simulink model "sst_llc_npc_inv"  (R2025b)
settings: Solver=ode23tb  StartTime=0.0  StopTime=simlength  FixedStep=tc  MaxStep=tc
values from neighbouring files (symbols this model uses):
  Adrso = eye(2) + Arso*ts_inv    [init_model.m]
  Aresd_max = eye(2) + Ares_max*ts_afe    [init_model.m]
  Aresd_min = eye(2) + Ares_min*ts_afe    [init_model.m]
  Aresd_nom = eye(2) + Ares_nom*ts_afe    [init_model.m]
  Bresd = Bres*ts_afe    [init_model.m]
  CFi_dc2 = 900e-6*4    (= 0.0036)    [init_model.m]
  Cresd = Cres    [init_model.m]
  Crso = [1 0]    [init_model.m]
  delta = 0.025    [init_model.m]
  fPWM_DAB = fPWM*4    (= 20000)    [init_model.m]
  fPWM_LLC_pu = 0.54    [init_model.m]
  freq = f_grid    [init_model.m]
  Iac_FS = I_phase_normalization_factor    [init_model.m]
  Idc_FS = max(Idab1_dc_nom,Idab2_dc_nom) * margin_factor    [init_model.m]
  iph_grid_pu_ref = 2.75    [init_model.m]
  ki_afe = 18    [init_model.m]
  ki_pll = 3140    [init_model.m]
  ki_rpi = 18    [init_model.m]
  kp_afe = 0.25    [init_model.m]
  kp_pll = 314    [init_model.m]
  kp_rpi = 0.25    [init_model.m]
  Ldrso = acker(Adrso',Crso',polesdrso)'    [init_model.m]
  LFu1_AFE = 0.33e-3    (= 0.00033)    [init_model.m]
  n_modules = 2    [init_model.m]
  RLFu1_AFE = 157*0.05*LFu1_AFE    (= 0.0025905)    [init_model.m]
  tc = ts_dab/100    (= 5e-07)    [init_model.m]
  ts_afe = 1/fPWM_AFE    (= 0.0002)    [init_model.m]
  ts_dab = 1/fPWM_DAB    (= 5e-05)    [init_model.m]
  ts_inv = 1/fPWM_INV    (= 0.0002)    [init_model.m]
  Vac_FS = V_phase_normalization_factor    [init_model.m]
  Vdab2_dc_nom = 750    [init_model.m]
  Vdc_FS = max(Vdab1_dc_nom,Vdab2_dc_nom) * margin_factor    [init_model.m]
undefined symbols (not defined in the file or in its folder): f_grid, Ld2_trafo, omega_grid_nom, Rd2_trafo, V_phase_normalization_factor
libraries: fl_lib x67, nesl_utility x39, full_bridge_mosfet_based_with_thermal_model x4, full_bridge_mosfet_based_with_thermal_model_zvs x4, pi_ctrl x4, discrete_time_low_pass_filter x4, full_bridge_three_level_npc_ideal_switch_based_model x3, single_phase_transformer x2, moving_average_filter x2, resonant_llc_modulator x2, full_bridge_ideal_switch x2, dclink_for_three_levels x2
(part 1 of 4)
settings Model: SimulationMode=accelerator  Creator=LTNBDA  LastModifiedBy=dbagn
settings SolverCC: ZeroCrossControl=EnableAll  ZeroCrossAlgorithm=Adaptive  AlgebraicLoopSolver=TrustRegion  SolverResetMethod=Robust  AutoInsertRateTranBlk=on
settings DataIOCC: LimitDataPoints=on  MaxDataPoints=1  SaveFormat=Array  SignalLoggingSaveFormat=ModelDataLogs  SaveOutput=off  SignalLogging=off  DSMLogging=off  SaveTime=off  ReturnWorkspaceOutputs=off
settings OptimizationCC: ExpressionDepthLimit=2147483647.0  InitFltsAndDblsToZero=on  EfficientMapNaN2IntZero=off  LifeSpan=inf
settings DebuggingCC: SaveWithParameterizedLinksMsg=none  UnderspecifiedInitializationDetection=Classic  MergeDetectMultiDrivingBlocksExec=none  SignalResolutionControl=TryResolveAllWithWarning  SolverPrmCheckMsg=warning  MultiTaskDSMMsg=warning  MultiTaskCondExecSysMsg=none  MultiTaskRateTransMsg=warning  FcnCallInpInsideContextMsg=warning  StateNameClashWarn=warning  SFUnexpectedBacktrackingDiag=warning  SFNoUnconditionalDefaultTransitionDiag=warning  ArithmeticOperatorsInVariantConditions=warning
settings HardwareCC: ProdBitPerLong=64.0  ProdLargestAtomicFloat=None  ProdIntDivRoundTo=Undefined  ProdEndianess=Unspecified  ProdHWDeviceType=Generic->64-bit Embedded Processor (LP64)  TargetBitPerPointer=64.0  TargetBitPerSizeT=64.0  TargetBitPerPtrDiffT=64.0  TargetLongLongMode=on  TargetIntDivRoundTo=Zero  TargetEndianess=LittleEndian  TargetWordSize=64.0  TargetHWDeviceType=MATLAB Host  ProdEqTarget=off
settings ModelReferenceCC: EnableRefExpFcnMdlSchedulingChecks=on  PropagateSignalLabelsOutOfModel=off
settings SFSimCC: SimUseLocalCustomCode=off  CustomCodeUndefinedFunction=UseInterfaceOnly
settings SFSimCC: SimCustomHeaderCode=|
  | #include "rpi.h"
  | #include "rpi_simulink.h"
  | #include "mavgflt.h"
  | #include "mavgflt_simulink.h"
  | #include "bemf_obsv.h"
  | #include "bemf_obsv_simulink.h"
  | #include "bemf_obsv_load_est.h"
  | #include "bemf_obsv_load_est_simulink.h"
  | #include "dqvector_pi.h"
  | #include "dqvector_pi_simulink.h"
  | #include "sv_pwm_simulink.h"
  | #include "sv_pwm.h"
  | #include "first_harmonic_tracker.h"
  | #include "first_harmonic_tracker_simulink.h"
  | #include "dqpll_thyr.h"
  | #include "dqpll_thyr_simulink.h"
  | #include "dqpll_grid.h"
  | #include "dqpll_grid_simulink.h"
settings SFSimCC: SimUserSources=|
  | "mavgflt_simulink.c"
  | "mavgflt.c"
  | "bemf_obsv_simulink.c"
  | "bemf_obsv.c"
  | "bemf_obsv_load_est_simulink.c"
  | "bemf_obsv_load_est.c"
  | "dqvector_pi.c"
  | "dqvector_pi_simulink.c"
  | "sv_pwm_simulink.c"
  | "sv_pwm.c"
  | "first_harmonic_tracker_simulink.c"
  | "first_harmonic_tracker.c"
  | "dqpll_thyr_simulink.c"
  | "dqpll_thyr.c"
  | "dqpll_grid_simulink.c"
  | "dqpll_grid.c"
  | "rpi_simulink.c"
  | "rpi.c"
settings SFSimCC: SimUserIncludeDirs=|
  | include
  | src
settings RTWCC: RTWUseLocalCustomCode=off  GPUComputeCapability=3.5
settings CodeAppCC: MaxIdLength=128.0  StateflowObjectComments=on
settings GRTTargetCC: TargetLangStandard=C89/C90 (ANSI)  CombineOutputUpdateFcns=off  GRTInterface=on
settings ConfigComp: CovMetricSettings=dw  CovSaveCumulativeToWorkspaceVar=on  CovSaveSingleToWorkspaceVar=on  CovExternalEMLEnable=off
settings SimscapeCC: SimscapeNormalizeSystem=off

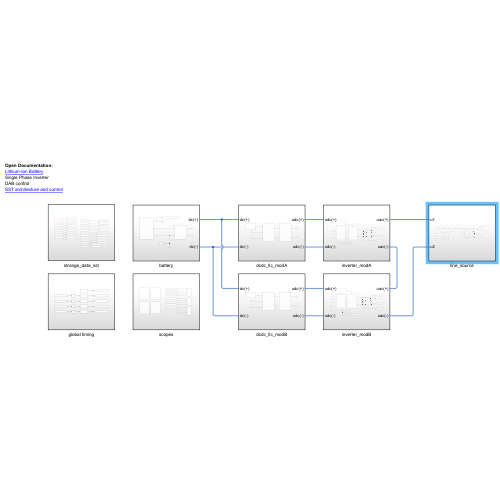
[thumbnail: Simulink's stored preview of the top-level diagram]
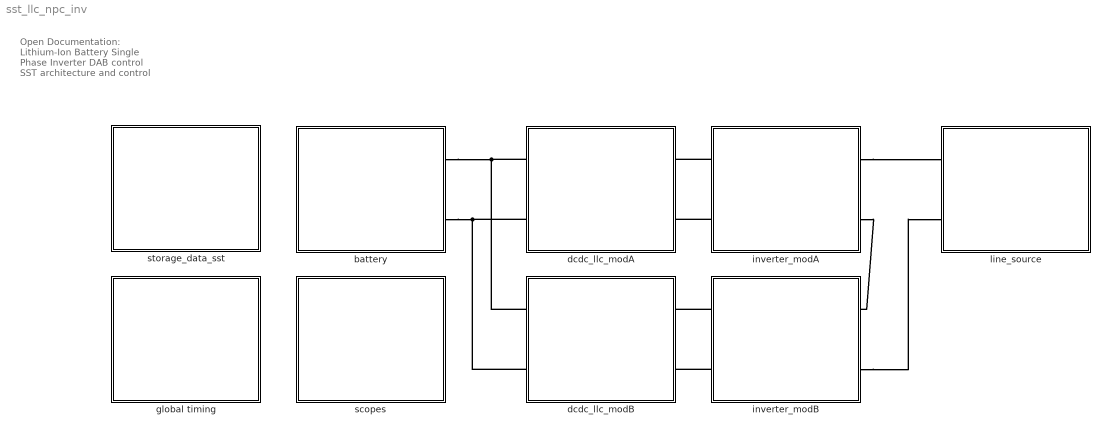
== system sst_llc_npc_inv ==
  note: Open Documentation:
      | Lithium-Ion Battery
      | Single Phase Inverter
      | DAB control
      | SST architecture and control
  battery : Subsystem
  dcdc_llc_modA : Subsystem
  dcdc_llc_modB : Subsystem
  global timing : Subsystem
  inverter_modA : Subsystem
  inverter_modB : Subsystem
  line_source : Subsystem
  scopes : Subsystem
  storage_data_sst : Subsystem
  connections:
  inverter_modA/LConn2 -- dcdc_llc_modA/RConn2
  inverter_modA/LConn1 -- dcdc_llc_modA/RConn1
  battery/RConn1 -- dcdc_llc_modB/LConn1 -- dcdc_llc_modA/LConn1
  battery/RConn2 -- dcdc_llc_modB/LConn2 -- dcdc_llc_modA/LConn2
  inverter_modB/LConn1 -- dcdc_llc_modB/RConn1
  inverter_modB/LConn2 -- dcdc_llc_modB/RConn2
  inverter_modA/RConn1 -- line_source/LConn1
  inverter_modA/RConn2 -- inverter_modB/RConn1
  inverter_modB/RConn2 -- line_source/LConn2

== system sst_llc_npc_inv/battery ==
  Electrical Reference1 : fl_lib/Electrical/Electrical Elements/Electrical Reference
  Solver Configuration : nesl_utility/Solver Configuration  PhysicalDomain=network_engine_domain  SubClassName=solver  LeftPortType=input  RightPortType=generic  Tones=[]  Harmonics=[]  SimulateNoise=off  Profile=off  UseLocalSampling=off  EnableSwitchedLinearOptims=on  FrequencyDomain=off  UseCCode=off  RelTol=0.001  AbsTol=0.001  MinStep=1e-09  ToWorkspace=off  RevertToSquareIcSolve=off  NumHomotopyIterations=100  PhasorMode=off  PhasorModeNumHarmonics=1  ConsistencySolver=NEWTON_FTOL  IndexReductionMethod=DerivativeReplacement  DoDC=on  ResidualTolerance=1e-09  ConsistencyTolSource=GLOBAL  ConsistencyAbsTol=0.001  ConsistencyRelTol=0.001  ConsistencyTolFactor=0.001  UseLocalSolver=on  LocalSolverChoice=NE_BACKWARD_EULER_ADVANCER  ResolveIndetEquations=on  FunctionEvalNumThread=1  LocalSolverSampleTime=tc  DoFixedCost=on  MaxNonlinIter=5  MaxModeIter=2  ComputeImpulses=off  ImpulseIterations=2  LinearAlgebra=auto  LinearAlgebraNumThread=0  EquationFormulation=NE_TIME_EF  DelaysMemoryBudget=1024  AutomaticFiltering=on  FilteringTimeConstant=0.001  PartitionStorageMethod=AS_NEEDED  PartitionMemoryBudget=1024  PartitionMethod=ROBUST  MultibodyUseLocalSolver=off  MultibodyLocalSolverChoice=ODE1  MultibodyLocalSolverSampleTime=0.001
  To Workspace14 : ToWorkspace  VariableName=battery_data  SampleTime=tc
      settings: MaxDataPoints=Nc
  litium ion battery : Scope
      settings: ActiveDisplayYMinimum=-797.80832786516225  ActiveDisplayYMaximum=1570.6184440426914  DataLoggingVariableName=ScopeData3
  litium_ion_battery : litium_ion_battery/litium_ion_battery  Q=Q  number_of_cells=number_of_cells  E_1=E_1  E0=E0  E1=E1  E2=E2  E3=E3  Elog=Elog  R0=R0  R1=R1  C1=C1  M=M  alpha=alpha  soc_init=0.85  ts_battery=ts_battery  q1Kalman=q1Kalman  q2Kalman=q2Kalman  q3Kalman=q3Kalman  rKalman=rKalman  tc=tc
  single_phase_ui_measure : Subsystem
  dc(+) : PMIOPort  Side=Right
  dc(-) : PMIOPort  Port=2  Side=Right
  wires:
  litium_ion_battery/1 -> To Workspace14/1, litium ion battery/1
  connections:
  litium_ion_battery/RConn2 -- single_phase_ui_measure/LConn2 -- Electrical Reference1/LConn1 -- Solver Configuration/RConn1
  single_phase_ui_measure/RConn1 -- dc(+)/RConn1
  single_phase_ui_measure/LConn1 -- litium_ion_battery/RConn1
  dc(-)/RConn1 -- single_phase_ui_measure/RConn2

== system sst_llc_npc_inv/dcdc_llc_modA ==
  dc/dc with galvanic isolation : Subsystem
  llc_ctrl : Subsystem
  ui_measure : Subsystem
  udc(+) : PMIOPort  Side=Right
  udc(-) : PMIOPort  Port=2  Side=Right
  dc(+) : PMIOPort  Port=3  Side=Left
  dc(-) : PMIOPort  Port=4  Side=Left
  wires:
  llc_ctrl/1(dab_gate_cmds) -> dc/dc with galvanic isolation/1(dab_gate_cmds)
  connections:
  dc/dc with galvanic isolation/RConn1 -- ui_measure/LConn1
  dc/dc with galvanic isolation/RConn2 -- ui_measure/LConn2
  udc(+)/RConn1 -- ui_measure/RConn1
  udc(-)/RConn1 -- ui_measure/RConn2
  dc(-)/RConn1 -- dc/dc with galvanic isolation/LConn2
  dc(+)/RConn1 -- dc/dc with galvanic isolation/LConn1

== system sst_llc_npc_inv/dcdc_llc_modB ==
  dc/dc with galvanic isolation : Subsystem
  llc_ctrl : Subsystem
  ui_measure : Subsystem
  udc(+) : PMIOPort  Side=Right
  udc(-) : PMIOPort  Port=2  Side=Right
  dc(+) : PMIOPort  Port=3  Side=Left
  dc(-) : PMIOPort  Port=4  Side=Left
  wires:
  llc_ctrl/1(dab_gate_cmds) -> dc/dc with galvanic isolation/1(dab_gate_cmds)
  connections:
  dc(+)/RConn1 -- dc/dc with galvanic isolation/LConn1
  dc(-)/RConn1 -- dc/dc with galvanic isolation/LConn2
  udc(-)/RConn1 -- ui_measure/RConn2
  udc(+)/RConn1 -- ui_measure/RConn1
  dc/dc with galvanic isolation/RConn2 -- ui_measure/LConn2
  dc/dc with galvanic isolation/RConn1 -- ui_measure/LConn1

== system sst_llc_npc_inv/global timing ==
  Unit Delay{,1..3} (4 alike) : UnitDelay  SampleTime=tc  HasFrameUpgradeWarning=on
  time_afe1 : Subsystem  mask{k=1}
      mask prompts: k "Time Gain"
      mask Display:
      | disp('time-gen');
      | port_label('input', 1, 'crt');
      | port_label('output', 1, 'tout');
  time_afe2 : Subsystem  mask{k=1}
      mask prompts: k "Time Gain"
      mask Display:
      | disp('time-gen');
      | port_label('input', 1, 'crt');
      | port_label('output', 1, 'tout');
  time_afe3 : Subsystem  mask{k=1}
      mask prompts: k "Time Gain"
      mask Display:
      | disp('time-gen');
      | port_label('output', 1, 'tout');
  time_inv1 : Subsystem  mask{k=1}
      mask prompts: k "Time Gain"
      mask Display:
      | disp('time-gen');
      | port_label('input', 1, 'crt');
      | port_label('output', 1, 'tout');
  time_inv2 : Subsystem  mask{k=1}
      mask prompts: k "Time Gain"
      mask Display:
      | disp('time-gen');
      | port_label('input', 1, 'crt');
      | port_label('output', 1, 'tout');
  tag scope: time_afe_module_1=global, time_afe_module_2=global, time_dab_module_1=global, time_dab_module_2=global, time_master=global
  wires:
  time_afe1/1(Out1) -> [time_afe_module_1]
  time_afe2/1(Out1) -> [time_dab_module_1]
  time_inv2/1(Out1) -> [time_dab_module_2]
  time_inv1/1(Out1) -> [time_afe_module_2]
  time_afe3/1(Out1) -> [time_master]
  [local_time_corr_afe1] -> Unit Delay/1
  Unit Delay/1 -> time_afe1/1(correction_time)
  [local_time_corr_dab1] -> Unit Delay1/1
  Unit Delay1/1 -> time_afe2/1(correction_time)
  [local_time_corr_afe2] -> Unit Delay2/1
  Unit Delay2/1 -> time_inv1/1(correction_time)
  Unit Delay3/1 -> time_inv2/1(correction_time)
  [local_time_corr_dab2] -> Unit Delay3/1

== system sst_llc_npc_inv/inverter_modA ==
  Bus Selector : BusSelector  OutputSignals=udc
  CFu_ac : fl_lib/Electrical/Electrical Elements/Capacitor  c=CFu_AFE F  r=RCFu_AFE Ohm  g=0 1/Ohm  i_specify=off  i_priority=None  i=0 A  i_nominal_specify=off  i_nominal_value=1  i_nominal_unit=A  v_specify=off  v_priority=None  v=0 V  v_nominal_specify=off  v_nominal_value=1  v_nominal_unit=V  vc_specify=off  vc_priority=High  vc=0 V  vc_nominal_specify=off  vc_nominal_value=1  vc_nominal_unit=V
  Current Sensor : fl_lib/Electrical/Electrical Sensors/Current Sensor
  Current Sensor1 : fl_lib/Electrical/Electrical Sensors/Current Sensor
  LFu_ac_1 : fl_lib/Electrical/Electrical Elements/Inductor  l=LFu1_AFE/2 H  r=RLFu1_AFE/2 Ohm  g=0 1/Ohm  i_specify=off  i_priority=None  i=0 A  i_nominal_specify=off  i_nominal_value=1  i_nominal_unit=A  v_specify=off  v_priority=None  v=0 V  v_nominal_specify=off  v_nominal_value=1  v_nominal_unit=V  i_L_specify=off  i_L_priority=High  i_L=0 A  i_L_nominal_specify=off  i_L_nominal_value=1  i_L_nominal_unit=A
  LFu_ac_2 : fl_lib/Electrical/Electrical Elements/Inductor  l=LFu1_AFE/2 H  r=RLFu1_AFE/2 Ohm  g=0 1/Ohm  i_specify=off  i_priority=None  i=0 A  i_nominal_specify=off  i_nominal_value=1  i_nominal_unit=A  v_specify=off  v_priority=None  v=0 V  v_nominal_specify=off  v_nominal_value=1  v_nominal_unit=V  i_L_specify=off  i_L_priority=High  i_L=0 A  i_L_nominal_specify=off  i_L_nominal_value=1  i_L_nominal_unit=A
  Open Circuit : fl_lib/Electrical/Electrical Elements/Open Circuit  v_specify=off  v_priority=None  v=0 V  v_nominal_specify=off  v_nominal_value=1  v_nominal_unit=V
  Resistor : fl_lib/Electrical/Electrical Elements/Resistor  R=10e3 Ohm  i_specify=off  i_priority=None  i=0 A  i_nominal_specify=off  i_nominal_value=1  i_nominal_unit=A  v_specify=off  v_priority=None  v=0 V  v_nominal_specify=off  v_nominal_value=1  v_nominal_unit=V
  Voltage Sensor1 : fl_lib/Electrical/Electrical Sensors/Voltage Sensor
  dclink : dclink_for_three_levels/dclink  Cdc1=CFi_dc2*2  Cdc2=CFi_dc2*2  Rudc_measure=107e3  Vdc_scale=Vdc_FS
  iph : nesl_utility/PS-Simulink Converter  PhysicalDomain=network_engine_domain  SubClassName=ps_output  LeftPortType=input  RightPortType=output  PseudoPeriodic=off  Frequencies=[]  VectorFormat=1-D array  Unit=A  AffineConversion=off
  single phase inverter : Subsystem
      settings: PortSchema="{\"entries\":[{\"content\":{\"sides\":[{\"content\":{\"connectorIds\":[\"LConn1\",\"LConn2\"]},\"type\":\"ConnectorPlacement.EquallySpacedRectSide\",\"uuid\":\"4fcf4fea-d38f-431b-8a91-be3ce9782faf\"},{\"content\":{\"connectorIds\":[\"RConn1\",\"RConn2\",\"RConn3\"],\"side\":\"RIGHT\"},\"type\":\"ConnectorPlacement.EquallySpacedRectSide\",\"uuid\":\"0aa56277-92e9-4e3b-84c7-43398254a4d8\"},{\"content\":{\"connectorIds\":[\"In1\"],\"side\":\"TOP\"},\"type\":\"ConnectorPlacement.EquallySpacedRectSide\",\"uuid\":\"5cd150dc-bcaf-4cd7-b2a8-3db203726730\"}]},\"type\":\"ConnectorPlacement.EquallySpacedConnector\",\"uuid\":\"bf8194c4-c327-4d40-bea4-f1e7617f80b4\"}],\"packageUris\":[\"http://schema.mathworks.com/mf0/Connector/R2020b\"],\"version\":\"1.0\"}"
  single phase inverter control1 : Subsystem
  uph1 : nesl_utility/PS-Simulink Converter  PhysicalDomain=network_engine_domain  SubClassName=ps_output  LeftPortType=input  RightPortType=output  PseudoPeriodic=off  Frequencies=[]  VectorFormat=1-D array  Unit=V  AffineConversion=off
  uph2 : nesl_utility/PS-Simulink Converter  PhysicalDomain=network_engine_domain  SubClassName=ps_output  LeftPortType=input  RightPortType=output  PseudoPeriodic=off  Frequencies=[]  VectorFormat=1-D array  Unit=A  AffineConversion=off
  uac(+) : PMIOPort  Side=Right
  uac(-) : PMIOPort  Port=2  Side=Right
  udc(+) : PMIOPort  Port=3  Side=Left
  udc(-) : PMIOPort  Port=4  Side=Left
  tag scope: CFu_ac_current_modA=global, dclink_inverter_modA=global, dclink_voltage_inverter_modA=global, inverter_current_output_modA=global, inverter_voltage_output_modA=global, u_ctrl_out_master=global
  wires:
  Bus Selector/1 -> [dclink_voltage_inverter_modA]  "<udc>"
  single phase inverter control1/1(gate_cmds) -> single phase inverter/1(gate_commands)
  iph/1 -> [inverter_current_output_modA]  "iph"
  uph1/1 -> [inverter_voltage_output_modA]  "uph"
  uph2/1 -> [CFu_ac_current_modA]
  single phase inverter control1/2(u_ctrl_out) -> [u_ctrl_out_master]
  dclink/1 -> [dclink_inverter_modA], Bus Selector/1
  connections:
  single phase inverter/LConn1 -- LFu_ac_1/LConn1
  single phase inverter/LConn2 -- LFu_ac_2/RConn1
  Voltage Sensor1/RConn1 -- uph1/LConn1
  Resistor/LConn1 -- Current Sensor/LConn1 -- Current Sensor1/LConn1 -- LFu_ac_1/RConn1
  iph/LConn1 -- Current Sensor/RConn1
  uac(+)/RConn1 -- Current Sensor/RConn2 -- Voltage Sensor1/LConn1
  LFu_ac_2/LConn1 -- uac(-)/RConn1 -- Voltage Sensor1/RConn2 -- Resistor/RConn1 -- CFu_ac/RConn1
  Current Sensor1/RConn2 -- CFu_ac/LConn1
  Current Sensor1/RConn1 -- uph2/LConn1
  single phase inverter/RConn1 -- dclink/LConn1
  single phase inverter/RConn2 -- dclink/LConn2
  single phase inverter/RConn3 -- dclink/LConn3
  udc(+)/RConn1 -- dclink/RConn1
  udc(-)/RConn1 -- dclink/RConn3
  Open Circuit/LConn1 -- dclink/RConn2

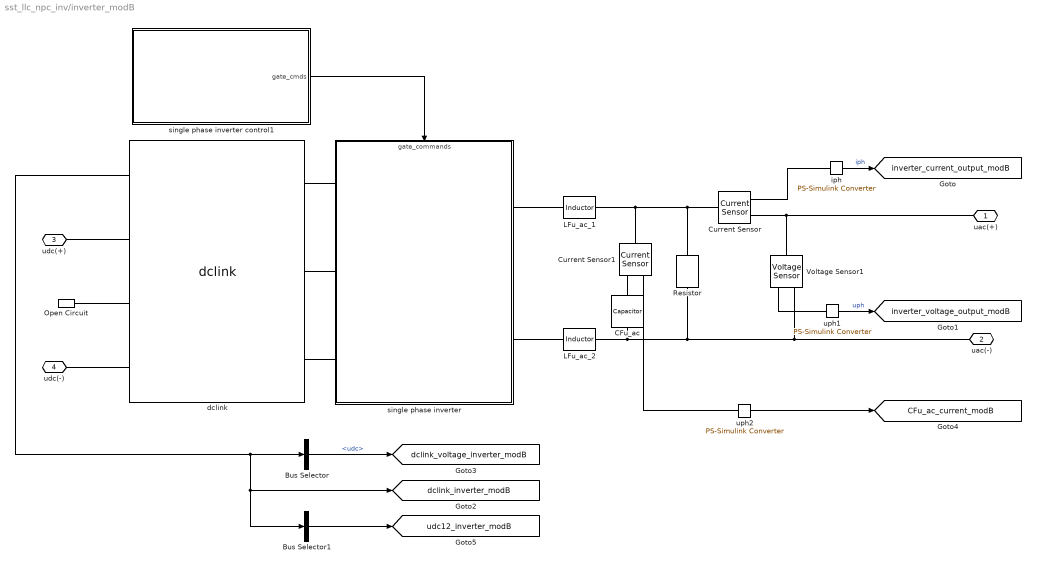
== system sst_llc_npc_inv/inverter_modB ==
  Bus Selector : BusSelector  OutputSignals=udc
  Bus Selector1 : BusSelector  OutputSignals=udc1,udc2  OutputAsBus=on
  CFu_ac : fl_lib/Electrical/Electrical Elements/Capacitor  c=CFu_AFE F  r=RCFu_AFE Ohm  g=0 1/Ohm  i_specify=off  i_priority=None  i=0 A  i_nominal_specify=off  i_nominal_value=1  i_nominal_unit=A  v_specify=off  v_priority=None  v=0 V  v_nominal_specify=off  v_nominal_value=1  v_nominal_unit=V  vc_specify=off  vc_priority=High  vc=0 V  vc_nominal_specify=off  vc_nominal_value=1  vc_nominal_unit=V
  Current Sensor : fl_lib/Electrical/Electrical Sensors/Current Sensor
  Current Sensor1 : fl_lib/Electrical/Electrical Sensors/Current Sensor
  LFu_ac_1 : fl_lib/Electrical/Electrical Elements/Inductor  l=LFu1_AFE/2 H  r=RLFu1_AFE/2 Ohm  g=0 1/Ohm  i_specify=off  i_priority=None  i=0 A  i_nominal_specify=off  i_nominal_value=1  i_nominal_unit=A  v_specify=off  v_priority=None  v=0 V  v_nominal_specify=off  v_nominal_value=1  v_nominal_unit=V  i_L_specify=off  i_L_priority=High  i_L=0 A  i_L_nominal_specify=off  i_L_nominal_value=1  i_L_nominal_unit=A
  LFu_ac_2 : fl_lib/Electrical/Electrical Elements/Inductor  l=LFu1_AFE/2 H  r=RLFu1_AFE/2 Ohm  g=0 1/Ohm  i_specify=off  i_priority=None  i=0 A  i_nominal_specify=off  i_nominal_value=1  i_nominal_unit=A  v_specify=off  v_priority=None  v=0 V  v_nominal_specify=off  v_nominal_value=1  v_nominal_unit=V  i_L_specify=off  i_L_priority=High  i_L=0 A  i_L_nominal_specify=off  i_L_nominal_value=1  i_L_nominal_unit=A
  Open Circuit : fl_lib/Electrical/Electrical Elements/Open Circuit  v_specify=off  v_priority=None  v=0 V  v_nominal_specify=off  v_nominal_value=1  v_nominal_unit=V
  Resistor : fl_lib/Electrical/Electrical Elements/Resistor  R=10e3 Ohm  i_specify=off  i_priority=None  i=0 A  i_nominal_specify=off  i_nominal_value=1  i_nominal_unit=A  v_specify=off  v_priority=None  v=0 V  v_nominal_specify=off  v_nominal_value=1  v_nominal_unit=V
  Voltage Sensor1 : fl_lib/Electrical/Electrical Sensors/Voltage Sensor
  dclink : dclink_for_three_levels/dclink  Cdc1=CFi_dc2*2  Cdc2=CFi_dc2*2  Rudc_measure=107e3  Vdc_scale=Vdc_FS
  iph : nesl_utility/PS-Simulink Converter  PhysicalDomain=network_engine_domain  SubClassName=ps_output  LeftPortType=input  RightPortType=output  PseudoPeriodic=off  Frequencies=[]  VectorFormat=1-D array  Unit=A  AffineConversion=off
  single phase inverter : Subsystem
      settings: PortSchema="{\"entries\":[{\"content\":{\"sides\":[{\"content\":{\"connectorIds\":[\"LConn1\",\"LConn2\"]},\"type\":\"ConnectorPlacement.EquallySpacedRectSide\",\"uuid\":\"4fcf4fea-d38f-431b-8a91-be3ce9782faf\"},{\"content\":{\"connectorIds\":[\"RConn1\",\"RConn2\",\"RConn3\"],\"side\":\"RIGHT\"},\"type\":\"ConnectorPlacement.EquallySpacedRectSide\",\"uuid\":\"0aa56277-92e9-4e3b-84c7-43398254a4d8\"},{\"content\":{\"connectorIds\":[\"In1\"],\"side\":\"TOP\"},\"type\":\"ConnectorPlacement.EquallySpacedRectSide\",\"uuid\":\"5cd150dc-bcaf-4cd7-b2a8-3db203726730\"}]},\"type\":\"ConnectorPlacement.EquallySpacedConnector\",\"uuid\":\"bf8194c4-c327-4d40-bea4-f1e7617f80b4\"}],\"packageUris\":[\"http://schema.mathworks.com/mf0/Connector/R2020b\"],\"version\":\"1.0\"}"
  single phase inverter control1 : Subsystem
  uph1 : nesl_utility/PS-Simulink Converter  PhysicalDomain=network_engine_domain  SubClassName=ps_output  LeftPortType=input  RightPortType=output  PseudoPeriodic=off  Frequencies=[]  VectorFormat=1-D array  Unit=V  AffineConversion=off
  uph2 : nesl_utility/PS-Simulink Converter  PhysicalDomain=network_engine_domain  SubClassName=ps_output  LeftPortType=input  RightPortType=output  PseudoPeriodic=off  Frequencies=[]  VectorFormat=1-D array  Unit=A  AffineConversion=off
  uac(+) : PMIOPort  Side=Right
  uac(-) : PMIOPort  Port=2  Side=Right
  udc(+) : PMIOPort  Port=3  Side=Left
  udc(-) : PMIOPort  Port=4  Side=Left
  tag scope: CFu_ac_current_modB=global, dclink_inverter_modB=global, dclink_voltage_inverter_modB=global, inverter_current_output_modB=global, inverter_voltage_output_modB=global, udc12_inverter_modB=global
  wires:
  uph2/1 -> [CFu_ac_current_modB]
  uph1/1 -> [inverter_voltage_output_modB]  "uph"
  iph/1 -> [inverter_current_output_modB]  "iph"
  single phase inverter control1/1(gate_cmds) -> single phase inverter/1(gate_commands)
  dclink/1 -> Bus Selector1/1, [dclink_inverter_modB], Bus Selector/1
  Bus Selector/1 -> [dclink_voltage_inverter_modB]  "<udc>"
  Bus Selector1/1 -> [udc12_inverter_modB]
  connections:
  Current Sensor1/RConn1 -- uph2/LConn1
  Current Sensor1/RConn2 -- CFu_ac/LConn1
  CFu_ac/RConn1 -- Resistor/RConn1 -- Voltage Sensor1/RConn2 -- uac(-)/RConn1 -- LFu_ac_2/LConn1
  Voltage Sensor1/LConn1 -- Current Sensor/RConn2 -- uac(+)/RConn1
  iph/LConn1 -- Current Sensor/RConn1
  LFu_ac_1/RConn1 -- Current Sensor1/LConn1 -- Current Sensor/LConn1 -- Resistor/LConn1
  Voltage Sensor1/RConn1 -- uph1/LConn1
  single phase inverter/LConn2 -- LFu_ac_2/RConn1
  LFu_ac_1/LConn1 -- single phase inverter/LConn1
  dclink/LConn1 -- single phase inverter/RConn1
  dclink/LConn2 -- single phase inverter/RConn2
  dclink/LConn3 -- single phase inverter/RConn3
  Open Circuit/LConn1 -- dclink/RConn2
  udc(+)/RConn1 -- dclink/RConn1
  udc(-)/RConn1 -- dclink/RConn3

== system sst_llc_npc_inv/line_source ==
  Controlled Voltage Source : fl_lib/Electrical/Electrical Sources/Controlled Voltage Source
  Controlled Voltage Source1 : fl_lib/Electrical/Electrical Sources/Controlled Voltage Source
  Cos : Trigonometry  Operator=cos
  Current Sensor : fl_lib/Electrical/Electrical Sensors/Current Sensor
  Electrical Reference : fl_lib/Electrical/Electrical Elements/Electrical Reference
  Gain : Gain  Gain=V_phase_normalization_factor
  Gain1 : Gain  Gain=n_modules
  Gain2 : Gain  Gain=1/2
  Ld_grid_1 : fl_lib/Electrical/Electrical Elements/Inductor  l=Ld2_trafo/2 H  r=Rd2_trafo/2 Ohm  g=0 1/Ohm  i_specify=off  i_priority=None  i=0 A  i_nominal_specify=off  i_nominal_value=1  i_nominal_unit=A  v_specify=off  v_priority=None  v=0 V  v_nominal_specify=off  v_nominal_value=1  v_nominal_unit=V  i_L_specify=off  i_L_priority=High  i_L=0 A  i_L_nominal_specify=off  i_L_nominal_value=1  i_L_nominal_unit=A
  Ld_grid_2 : fl_lib/Electrical/Electrical Elements/Inductor  l=Ld2_trafo/2 H  r=Rd2_trafo/2 Ohm  g=0 1/Ohm  i_specify=off  i_priority=None  i=0 A  i_nominal_specify=off  i_nominal_value=1  i_nominal_unit=A  v_specify=off  v_priority=None  v=0 V  v_nominal_specify=off  v_nominal_value=1  v_nominal_unit=V  i_L_specify=off  i_L_priority=High  i_L=0 A  i_L_nominal_specify=off  i_L_nominal_value=1  i_L_nominal_unit=A
  Simulink-PS Converter : nesl_utility/Simulink-PS Converter  PhysicalDomain=network_engine_domain  SubClassName=ps_input  LeftPortType=input  RightPortType=output  PseudoPeriodic=off  Frequencies=[]  NoiseDistribution=none  NoiseParameters=[]  Unit=1  AffineConversion=off  FilteringAndDerivatives=provide  SimscapeFilterOrder=1  InputFilterTimeConstant=0.001  UdotUserProvided=0
  Voltage Sensor2 : fl_lib/Electrical/Electrical Sensors/Voltage Sensor
  i_line : nesl_utility/PS-Simulink Converter  PhysicalDomain=network_engine_domain  SubClassName=ps_output  LeftPortType=input  RightPortType=output  PseudoPeriodic=off  Frequencies=[]  VectorFormat=1-D array  Unit=A  AffineConversion=off
  phase_gen : Subsystem
  phase_grid/pll : Scope  NumInputPorts=3
      settings: SampleTime=tc  ActiveDisplayYMinimum=-3.9269580058491287  ActiveDisplayYMaximum=3.9266955167607471
  u_line_source : nesl_utility/PS-Simulink Converter  PhysicalDomain=network_engine_domain  SubClassName=ps_output  LeftPortType=input  RightPortType=output  PseudoPeriodic=off  Frequencies=[]  VectorFormat=1-D array  Unit=V  AffineConversion=off
  u1 : PMIOPort  Side=Left
  u2 : PMIOPort  Port=2  Side=Left
  tag scope: ac_grid_current=global, ac_grid_voltage=global, phase_grid=global
  wires:
  phase_gen/1(phase_gen) -> Cos/1, [phase_grid]
  Cos/1 -> Gain1/1
  Gain/1 -> Gain2/1
  [phase_synch_modA] -> phase_grid/pll/1  "phase_synch_modA"
  [phase_grid] -> phase_grid/pll/2  "phase_grid"
  u_line_source/1 -> [ac_grid_voltage]  "u_line_source"
  Gain1/1 -> Gain/1
  [phase_synch_modB] -> phase_grid/pll/3  "phase_synch_modB"
  i_line/1 -> [ac_grid_current]  "u_line_source"
  Gain2/1 -> Simulink-PS Converter/1
  connections:
  Simulink-PS Converter/RConn1 -- Controlled Voltage Source1/RConn1 -- Controlled Voltage Source/RConn1
  Voltage Sensor2/RConn1 -- u_line_source/LConn1
  Ld_grid_1/RConn1 -- Current Sensor/LConn1 -- Voltage Sensor2/LConn1
  Controlled Voltage Source/RConn2 -- Controlled Voltage Source1/LConn1 -- Electrical Reference/LConn1
  Controlled Voltage Source/LConn1 -- Ld_grid_1/LConn1
  Current Sensor/RConn2 -- u1/RConn1
  Current Sensor/RConn1 -- i_line/LConn1
  u2/RConn1 -- Ld_grid_2/RConn1 -- Voltage Sensor2/RConn2
  Controlled Voltage Source1/RConn2 -- Ld_grid_2/LConn1

== system sst_llc_npc_inv/scopes ==
  DABs input current/voltage : Scope  NumInputPorts=4
      settings: ActiveDisplayString=3  ActiveDisplayYMinimum=-1  ActiveDisplayYMaximum=1  DataLoggingVariableName=ScopeData11
  DABs output current/voltage : Scope  NumInputPorts=4
      settings: ActiveDisplayString=3  ActiveDisplayYMinimum=-1181.3054875017851  ActiveDisplayYMaximum=884.19595504743074  DataLoggingVariableName=ScopeData9
  inverters current/voltage : Scope  NumInputPorts=4
      settings: ActiveDisplayString=3  ActiveDisplayYMinimum=-2204.1441129945752  ActiveDisplayYMaximum=1779.1998949653275
  scopes_dab_modA : Subsystem
  scopes_dab_modB : Subsystem
  scopes_inv_modA : Subsystem
  scopes_inv_modB : Subsystem
  wires:
  [inverter_current_output_modB] -> inverters current/voltage/3  "inverter_current_output_modB"
  [inverter_voltage_output_modB] -> inverters current/voltage/4  "inverter_voltage_output_modB"
  [inverter_voltage_output_modA] -> inverters current/voltage/2  "inverter_voltage_output_modA"
  [inverter_current_output_modA] -> inverters current/voltage/1  "inverter_current_output_modA"
  [dab_current_output_modA] -> DABs output current/voltage/1  "dab_current_output_modA"
  [dab_voltage_output_modA] -> DABs output current/voltage/2  "dab_voltage_output_modA"
  [dab_voltage_output_modB] -> DABs output current/voltage/4  "dab_voltage_output_modB"
  [dab_current_output_modB] -> DABs output current/voltage/3  "dab_current_output_modB"
  [dab_voltage_input_modB] -> DABs input current/voltage/3  "dab_voltage_input_modB"
  [dab_current_input_modB] -> DABs input current/voltage/4  "dab_current_input_modB"
  [dab_current_input_modA] -> DABs input current/voltage/2  "dab_current_input_modA"
  [dab_voltage_input_modA] -> DABs input current/voltage/1  "dab_voltage_input_modA"

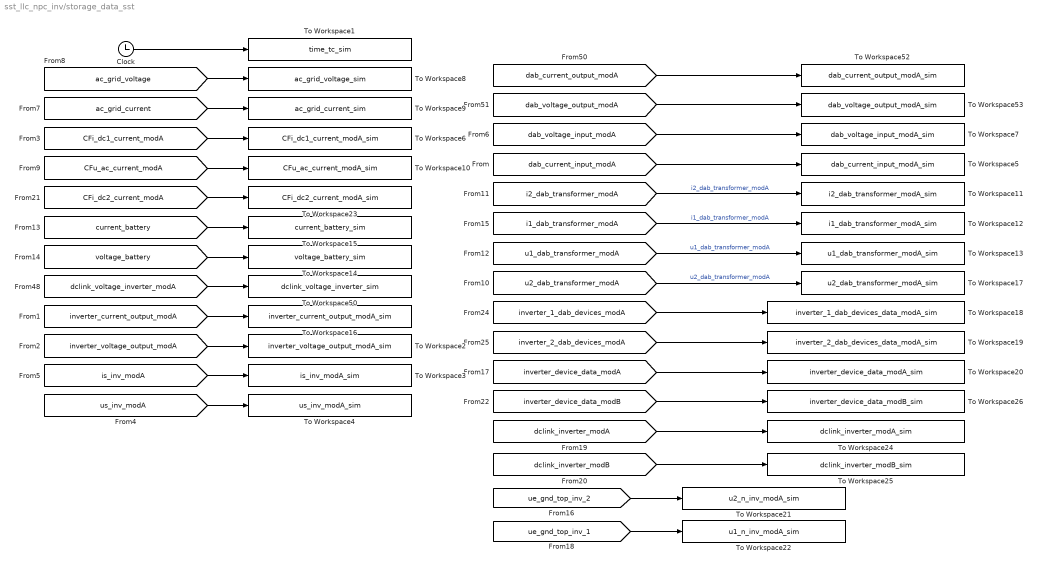
== system sst_llc_npc_inv/storage_data_sst ==
  Clock : Clock
  To Workspace1 : ToWorkspace  VariableName=time_tc_sim  SampleTime=tc
      settings: MaxDataPoints=Nc
  To Workspace10 : ToWorkspace  VariableName=CFu_ac_current_modA_sim  SampleTime=tc
      settings: MaxDataPoints=Nc
  To Workspace11 : ToWorkspace  VariableName=i2_dab_transformer_modA_sim  SampleTime=tc
      settings: MaxDataPoints=Nc
  To Workspace12 : ToWorkspace  VariableName=i1_dab_transformer_modA_sim  SampleTime=tc
      settings: MaxDataPoints=Nc
  To Workspace13 : ToWorkspace  VariableName=u1_dab_transformer_modA_sim  SampleTime=tc
      settings: MaxDataPoints=Nc
  To Workspace14 : ToWorkspace  VariableName=voltage_battery_sim  SampleTime=tc
      settings: MaxDataPoints=Nc
  To Workspace15 : ToWorkspace  VariableName=current_battery_sim  SampleTime=tc
      settings: MaxDataPoints=Nc
  To Workspace16 : ToWorkspace  VariableName=inverter_current_output_modA_sim  SampleTime=tc
      settings: MaxDataPoints=Nc
  To Workspace17 : ToWorkspace  VariableName=u2_dab_transformer_modA_sim  SampleTime=tc
      settings: MaxDataPoints=Nc
  To Workspace18 : ToWorkspace  VariableName=inverter_1_dab_devices_data_modA_sim  SampleTime=tc
      settings: MaxDataPoints=Nc
  To Workspace19 : ToWorkspace  VariableName=inverter_2_dab_devices_data_modA_sim  SampleTime=tc
      settings: MaxDataPoints=Nc
  To Workspace2 : ToWorkspace  VariableName=inverter_voltage_output_modA_sim  SampleTime=tc
      settings: MaxDataPoints=Nc
  To Workspace20 : ToWorkspace  VariableName=inverter_device_data_modA_sim  SampleTime=tc
      settings: MaxDataPoints=Nc
  To Workspace21 : ToWorkspace  VariableName=u2_n_inv_modA_sim  SampleTime=tc
      settings: MaxDataPoints=Nc
  To Workspace22 : ToWorkspace  VariableName=u1_n_inv_modA_sim  SampleTime=tc
      settings: MaxDataPoints=Nc
  To Workspace23 : ToWorkspace  VariableName=CFi_dc2_current_modA_sim  SampleTime=tc
      settings: MaxDataPoints=Nc
  To Workspace24 : ToWorkspace  VariableName=dclink_inverter_modA_sim  SampleTime=tc
      settings: MaxDataPoints=Nc
  To Workspace25 : ToWorkspace  VariableName=dclink_inverter_modB_sim  SampleTime=tc
      settings: MaxDataPoints=Nc
  To Workspace26 : ToWorkspace  VariableName=inverter_device_data_modB_sim  SampleTime=tc
      settings: MaxDataPoints=Nc
  To Workspace3 : ToWorkspace  VariableName=is_inv_modA_sim  SampleTime=tc
      settings: MaxDataPoints=Nc
  To Workspace4 : ToWorkspace  VariableName=us_inv_modA_sim  SampleTime=tc
      settings: MaxDataPoints=Nc
  To Workspace5 : ToWorkspace  VariableName=dab_current_input_modA_sim  SampleTime=tc
      settings: MaxDataPoints=Nc
  To Workspace50 : ToWorkspace  VariableName=dclink_voltage_inverter_sim  SampleTime=tc
      settings: MaxDataPoints=Nc
  To Workspace52 : ToWorkspace  VariableName=dab_current_output_modA_sim  SampleTime=tc
      settings: MaxDataPoints=Nc
  To Workspace53 : ToWorkspace  VariableName=dab_voltage_output_modA_sim  SampleTime=tc
      settings: MaxDataPoints=Nc
  To Workspace6 : ToWorkspace  VariableName=CFi_dc1_current_modA_sim  SampleTime=tc
      settings: MaxDataPoints=Nc
  To Workspace7 : ToWorkspace  VariableName=dab_voltage_input_modA_sim  SampleTime=tc
      settings: MaxDataPoints=Nc
  To Workspace8 : ToWorkspace  VariableName=ac_grid_voltage_sim  SampleTime=tc
      settings: MaxDataPoints=Nc
  To Workspace9 : ToWorkspace  VariableName=ac_grid_current_sim  SampleTime=tc
      settings: MaxDataPoints=Nc
  wires:
  Clock/1 -> To Workspace1/1
  [inverter_current_output_modA] -> To Workspace16/1
  [inverter_voltage_output_modA] -> To Workspace2/1
  [is_inv_modA] -> To Workspace3/1
  [us_inv_modA] -> To Workspace4/1
  [CFi_dc1_current_modA] -> To Workspace6/1
  [dab_voltage_input_modA] -> To Workspace7/1
  [CFu_ac_current_modA] -> To Workspace10/1
  [voltage_battery] -> To Workspace14/1
  [current_battery] -> To Workspace15/1
  [CFi_dc2_current_modA] -> To Workspace23/1
  [dclink_voltage_inverter_modA] -> To Workspace50/1
  [dab_voltage_output_modA] -> To Workspace53/1
  [dab_current_output_modA] -> To Workspace52/1
  [ac_grid_voltage] -> To Workspace8/1
  [ac_grid_current] -> To Workspace9/1
  [dab_current_input_modA] -> To Workspace5/1
  [i2_dab_transformer_modA] -> To Workspace11/1  "i2_dab_transformer_modA"
  [i1_dab_transformer_modA] -> To Workspace12/1  "i1_dab_transformer_modA"
  [u1_dab_transformer_modA] -> To Workspace13/1  "u1_dab_transformer_modA"
  [u2_dab_transformer_modA] -> To Workspace17/1  "u2_dab_transformer_modA"
  [inverter_1_dab_devices_modA] -> To Workspace18/1
  [inverter_2_dab_devices_modA] -> To Workspace19/1
  [inverter_device_data_modA] -> To Workspace20/1
  [dclink_inverter_modA] -> To Workspace24/1
  [dclink_inverter_modB] -> To Workspace25/1
  [inverter_device_data_modB] -> To Workspace26/1
  [ue_gnd_top_inv_2] -> To Workspace21/1
  [ue_gnd_top_inv_1] -> To Workspace22/1

== system sst_llc_npc_inv/battery/single_phase_ui_measure ==
  Bus Creator : BusCreator  Inputs=2
  Current Sensor : fl_lib/Electrical/Electrical Sensors/Current Sensor
  Selector : Selector  InputPortWidth=2  IndexOptions=Index vector (dialog)  Indices=2  OutputSizes=1
  Selector1 : Selector  InputPortWidth=2  IndexOptions=Index vector (dialog)  Indices=1  OutputSizes=1
  Voltage Sensor : fl_lib/Electrical/Electrical Sensors/Voltage Sensor
  dab input modA : Scope  NumInputPorts=2
      settings: SampleTime=tc  ActiveDisplayYMinimum=-359.9383171902324  ActiveDisplayYMaximum=-189.30707708261582  DataLoggingVariableName=ScopeData2
  iph : nesl_utility/PS-Simulink Converter  PhysicalDomain=network_engine_domain  SubClassName=ps_output  LeftPortType=input  RightPortType=output  PseudoPeriodic=off  Frequencies=[]  VectorFormat=1-D array  Unit=A  AffineConversion=off
  uph : nesl_utility/PS-Simulink Converter  PhysicalDomain=network_engine_domain  SubClassName=ps_output  LeftPortType=input  RightPortType=output  PseudoPeriodic=off  Frequencies=[]  VectorFormat=1-D array  Unit=V  AffineConversion=off
  Udc(+) : PMIOPort  Side=Left
  udc(+) : PMIOPort  Port=2  Side=Right
  Udc(-) : PMIOPort  Port=3  Side=Left
  udc(-) : PMIOPort  Port=4  Side=Right
  tag scope: current_battery=global, voltage_battery=global
  wires:
  Bus Creator/1 -> Selector/1, Selector1/1  "ui_data"
  iph/1 -> Bus Creator/1  "iph"
  uph/1 -> Bus Creator/2  "uph"
  Selector1/1 -> [current_battery], dab input modA/1  "current_battery"
  Selector/1 -> dab input modA/2, [voltage_battery]  "voltage_battery"
  connections:
  iph/LConn1 -- Current Sensor/RConn1
  Voltage Sensor/LConn1 -- Current Sensor/LConn1 -- Udc(+)/RConn1
  Current Sensor/RConn2 -- udc(+)/RConn1
  Voltage Sensor/RConn1 -- uph/LConn1
  Voltage Sensor/RConn2 -- Udc(-)/RConn1 -- udc(-)/RConn1

== system sst_llc_npc_inv/dcdc_llc_modA/dc//dc with galvanic isolation ==
  dab_gate_cmds : Inport
  Bus Selector : BusSelector  OutputSignals=full_bridge1.gate_cmd_Q1,full_bridge1.gate_cmd_Q2,full_bridge1.gate_cmd_Q3,full_bridge1.gate_cmd_Q4  OutputAsBus=on
  Bus Selector1 : BusSelector  OutputSignals=full_bridge2.gate_cmd_Q1,full_bridge2.gate_cmd_Q2,full_bridge2.gate_cmd_Q3,full_bridge2.gate_cmd_Q4  OutputAsBus=on
  CFi_dc1 : fl_lib/Electrical/Electrical Elements/Capacitor  c=CFi_dc1 F  r=RCFi_dc1_internal Ohm  g=0 1/Ohm  i_specify=off  i_priority=None  i=0 A  i_nominal_specify=off  i_nominal_value=1  i_nominal_unit=A  v_specify=off  v_priority=None  v=0 V  v_nominal_specify=off  v_nominal_value=1  v_nominal_unit=V  vc_specify=off  vc_priority=High  vc=0 V  vc_nominal_specify=off  vc_nominal_value=1  vc_nominal_unit=V
  Current Sensor : fl_lib/Electrical/Electrical Sensors/Current Sensor
  Current Sensor2 : fl_lib/Electrical/Electrical Sensors/Current Sensor
  LFi_dc : fl_lib/Electrical/Electrical Elements/Inductor  l=LFi_dc H  r=RLFi_dc Ohm  g=1e-9 1/Ohm  i_specify=off  i_priority=None  i=0 A  i_nominal_specify=off  i_nominal_value=1  i_nominal_unit=A  v_specify=off  v_priority=None  v=0 V  v_nominal_specify=off  v_nominal_value=1  v_nominal_unit=V  i_L_specify=off  i_L_priority=High  i_L=0 A  i_L_nominal_specify=off  i_L_nominal_value=1  i_L_nominal_unit=A
  PS-Simulink Converter1 : nesl_utility/PS-Simulink Converter  PhysicalDomain=network_engine_domain  SubClassName=ps_output  LeftPortType=input  RightPortType=output  PseudoPeriodic=off  Frequencies=[]  VectorFormat=1-D array  Unit=A  AffineConversion=on
  PS-Simulink Converter4 : nesl_utility/PS-Simulink Converter  PhysicalDomain=network_engine_domain  SubClassName=ps_output  LeftPortType=input  RightPortType=output  PseudoPeriodic=off  Frequencies=[]  VectorFormat=1-D array  Unit=V  AffineConversion=on
  PS-Simulink Converter6 : nesl_utility/PS-Simulink Converter  PhysicalDomain=network_engine_domain  SubClassName=ps_output  LeftPortType=input  RightPortType=output  PseudoPeriodic=off  Frequencies=[]  VectorFormat=1-D array  Unit=A  AffineConversion=on
  Voltage Sensor : fl_lib/Electrical/Electrical Sensors/Voltage Sensor
  full-bridge 1 : Subsystem
      settings: PortSchema="{\"entries\":[{\"content\":{\"sides\":[{\"content\":{\"connectorIds\":[\"LConn1\",\"LConn2\"]},\"type\":\"ConnectorPlacement.EquallySpacedRectSide\",\"uuid\":\"c872503a-61af-4937-bdf2-4de4f8645573\"},{\"content\":{\"connectorIds\":[\"RConn1\",\"RConn2\"],\"side\":\"RIGHT\"},\"type\":\"ConnectorPlacement.EquallySpacedRectSide\",\"uuid\":\"3b83f060-86a2-4569-84b5-d9f7c0485347\"},{\"content\":{\"connectorIds\":[\"In1\"],\"side\":\"TOP\"},\"type\":\"ConnectorPlacement.EquallySpacedRectSide\",\"uuid\":\"bf191d46-ce71-4d15-9dd0-24cc57253577\"}]},\"type\":\"ConnectorPlacement.EquallySpacedConnector\",\"uuid\":\"1b28ceee-25d0-45ae-a3c4-c2563f0d63ba\"}],\"packageUris\":[\"http://schema.mathworks.com/mf0/Connector/R2020b\"],\"version\":\"1.0\"}"
  full-bridge 2 : Subsystem
      settings: PortSchema="{\"entries\":[{\"content\":{\"sides\":[{\"content\":{\"connectorIds\":[\"LConn1\",\"LConn2\"]},\"type\":\"ConnectorPlacement.EquallySpacedRectSide\",\"uuid\":\"c872503a-61af-4937-bdf2-4de4f8645573\"},{\"content\":{\"connectorIds\":[\"RConn1\",\"RConn2\"],\"side\":\"RIGHT\"},\"type\":\"ConnectorPlacement.EquallySpacedRectSide\",\"uuid\":\"3b83f060-86a2-4569-84b5-d9f7c0485347\"},{\"content\":{\"connectorIds\":[\"In1\"],\"side\":\"TOP\"},\"type\":\"ConnectorPlacement.EquallySpacedRectSide\",\"uuid\":\"bf191d46-ce71-4d15-9dd0-24cc57253577\"}]},\"type\":\"ConnectorPlacement.EquallySpacedConnector\",\"uuid\":\"1b28ceee-25d0-45ae-a3c4-c2563f0d63ba\"}],\"packageUris\":[\"http://schema.mathworks.com/mf0/Connector/R2020b\"],\"version\":\"1.0\"}"
  single_phase_dab_transformer : Subsystem
  Udc(+) : PMIOPort  Side=Left
  udc(+) : PMIOPort  Port=2  Side=Right
  Udc(-) : PMIOPort  Port=3  Side=Left
  udc(-) : PMIOPort  Port=4  Side=Right
  tag scope: CFi_dc1_current_modA=global, dab_current_input_modA=global, dab_voltage_input_modA=global
  wires:
  PS-Simulink Converter1/1 -> [CFi_dc1_current_modA]  "CFi_dc_curren"
  PS-Simulink Converter4/1 -> [dab_voltage_input_modA]  "udc1_dab_modA"
  PS-Simulink Converter6/1 -> [dab_current_input_modA]  "idc"
  dab_gate_cmds/1 -> Bus Selector/1, Bus Selector1/1
  Bus Selector/1 -> full-bridge 1/1(gate_commands)
  Bus Selector1/1 -> full-bridge 2/1(gate_commands)
  connections:
  full-bridge 1/LConn2 -- single_phase_dab_transformer/LConn2
  CFi_dc1/LConn1 -- full-bridge 1/RConn1 -- Voltage Sensor/LConn1 -- LFi_dc/RConn1
  Current Sensor/RConn2 -- full-bridge 1/RConn2 -- Voltage Sensor/RConn2 -- Udc(-)/RConn1
  Current Sensor/LConn1 -- CFi_dc1/RConn1
  Current Sensor/RConn1 -- PS-Simulink Converter1/LConn1
  PS-Simulink Converter4/LConn1 -- Voltage Sensor/RConn1
  full-bridge 1/LConn1 -- single_phase_dab_transformer/LConn1
  full-bridge 2/RConn1 -- udc(+)/RConn1
  full-bridge 2/RConn2 -- udc(-)/RConn1
  Current Sensor2/RConn2 -- LFi_dc/LConn1
  Udc(+)/RConn1 -- Current Sensor2/LConn1
  Current Sensor2/RConn1 -- PS-Simulink Converter6/LConn1
  full-bridge 2/LConn1 -- single_phase_dab_transformer/RConn1
  full-bridge 2/LConn2 -- single_phase_dab_transformer/RConn2

== system sst_llc_npc_inv/dcdc_llc_modA/llc_ctrl ==
  dab_voltage&current_controllers : Subsystem
  modulator : Subsystem
  references : Subsystem
  sampling_i_filter1 : Subsystem
  sampling_v_filter1 : Subsystem
  sampling_v_filter2 : Subsystem
  dab_gate_cmds : Outport
  wires:
  references/1(vout_ref) -> sampling_v_filter2/1(in)
  sampling_v_filter2/1(out_pu) -> dab_voltage&current_controllers/3(dab_voltage_output pu_reference)  "dab_voltage_output_pu_reference"
  sampling_v_filter1/1(out_pu) -> dab_voltage&current_controllers/2(dab_voltage_output_pu)  "dab_voltage_output_pu"
  sampling_i_filter1/1(out_pu) -> dab_voltage&current_controllers/1(dab_current_input_pu)  "dab_current_input_pu"
  [dab_current_input_modA] -> sampling_i_filter1/1(in)
  [dab_voltage_output_modA] -> sampling_v_filter1/1(in)
  [TRGO_DCDC_1] -> dab_voltage&current_controllers/Trigger
  modulator/1(dab_gate_cmds) -> dab_gate_cmds/1
  [time_dab_module_1] -> dab_voltage&current_controllers/4(time_dab_module_1)  "time_dab_module_1"
  dab_voltage&current_controllers/1(freq_pu) -> modulator/1(freq_pu)
  dab_voltage&current_controllers/2(phase_disp) -> modulator/2(phase_displacement)

== system sst_llc_npc_inv/dcdc_llc_modA/ui_measure ==
  Bus Creator : BusCreator  Inputs=2
  Current Sensor : fl_lib/Electrical/Electrical Sensors/Current Sensor
  Selector : Selector  InputPortWidth=2  IndexOptions=Index vector (dialog)  Indices=2  OutputSizes=1
  Selector1 : Selector  InputPortWidth=2  IndexOptions=Index vector (dialog)  Indices=1  OutputSizes=1
  Voltage Sensor : fl_lib/Electrical/Electrical Sensors/Voltage Sensor
  iph : nesl_utility/PS-Simulink Converter  PhysicalDomain=network_engine_domain  SubClassName=ps_output  LeftPortType=input  RightPortType=output  PseudoPeriodic=off  Frequencies=[]  VectorFormat=1-D array  Unit=A  AffineConversion=off
  uph : nesl_utility/PS-Simulink Converter  PhysicalDomain=network_engine_domain  SubClassName=ps_output  LeftPortType=input  RightPortType=output  PseudoPeriodic=off  Frequencies=[]  VectorFormat=1-D array  Unit=V  AffineConversion=off
  Udc(+) : PMIOPort  Side=Left
  udc(+) : PMIOPort  Port=2  Side=Right
  Udc(-) : PMIOPort  Port=3  Side=Left
  udc(-) : PMIOPort  Port=4  Side=Right
  tag scope: dab_current_output_modA=global, dab_voltage_output_modA=global
  wires:
  Selector1/1 -> [dab_current_output_modA]
  Selector/1 -> [dab_voltage_output_modA]
  Bus Creator/1 -> Selector/1, Selector1/1  "ui_data"
  iph/1 -> Bus Creator/1  "iph"
  uph/1 -> Bus Creator/2  "uph"
  connections:
  iph/LConn1 -- Current Sensor/RConn1
  Voltage Sensor/LConn1 -- Current Sensor/LConn1 -- Udc(+)/RConn1
  Current Sensor/RConn2 -- udc(+)/RConn1
  Voltage Sensor/RConn1 -- uph/LConn1
  Voltage Sensor/RConn2 -- Udc(-)/RConn1 -- udc(-)/RConn1

== system sst_llc_npc_inv/dcdc_llc_modB/dc//dc with galvanic isolation ==
  dab_gate_cmds : Inport
  Bus Selector : BusSelector  OutputSignals=full_bridge1.gate_cmd_Q1,full_bridge1.gate_cmd_Q2,full_bridge1.gate_cmd_Q3,full_bridge1.gate_cmd_Q4  OutputAsBus=on
  Bus Selector1 : BusSelector  OutputSignals=full_bridge2.gate_cmd_Q1,full_bridge2.gate_cmd_Q2,full_bridge2.gate_cmd_Q3,full_bridge2.gate_cmd_Q4  OutputAsBus=on
  CFi_dc1 : fl_lib/Electrical/Electrical Elements/Capacitor  c=CFi_dc1 F  r=RCFi_dc1_internal Ohm  g=0 1/Ohm  i_specify=off  i_priority=None  i=0 A  i_nominal_specify=off  i_nominal_value=1  i_nominal_unit=A  v_specify=off  v_priority=None  v=0 V  v_nominal_specify=off  v_nominal_value=1  v_nominal_unit=V  vc_specify=off  vc_priority=High  vc=0 V  vc_nominal_specify=off  vc_nominal_value=1  vc_nominal_unit=V
  Current Sensor : fl_lib/Electrical/Electrical Sensors/Current Sensor
  Current Sensor2 : fl_lib/Electrical/Electrical Sensors/Current Sensor
  LFi_dc : fl_lib/Electrical/Electrical Elements/Inductor  l=LFi_dc H  r=RLFi_dc Ohm  g=1e-9 1/Ohm  i_specify=off  i_priority=None  i=0 A  i_nominal_specify=off  i_nominal_value=1  i_nominal_unit=A  v_specify=off  v_priority=None  v=0 V  v_nominal_specify=off  v_nominal_value=1  v_nominal_unit=V  i_L_specify=off  i_L_priority=High  i_L=0 A  i_L_nominal_specify=off  i_L_nominal_value=1  i_L_nominal_unit=A
  PS-Simulink Converter1 : nesl_utility/PS-Simulink Converter  PhysicalDomain=network_engine_domain  SubClassName=ps_output  LeftPortType=input  RightPortType=output  PseudoPeriodic=off  Frequencies=[]  VectorFormat=1-D array  Unit=A  AffineConversion=on
  PS-Simulink Converter4 : nesl_utility/PS-Simulink Converter  PhysicalDomain=network_engine_domain  SubClassName=ps_output  LeftPortType=input  RightPortType=output  PseudoPeriodic=off  Frequencies=[]  VectorFormat=1-D array  Unit=V  AffineConversion=on
  PS-Simulink Converter6 : nesl_utility/PS-Simulink Converter  PhysicalDomain=network_engine_domain  SubClassName=ps_output  LeftPortType=input  RightPortType=output  PseudoPeriodic=off  Frequencies=[]  VectorFormat=1-D array  Unit=A  AffineConversion=on
  Voltage Sensor : fl_lib/Electrical/Electrical Sensors/Voltage Sensor
  full-bridge 1 : Subsystem
      settings: PortSchema="{\"entries\":[{\"content\":{\"sides\":[{\"content\":{\"connectorIds\":[\"LConn1\",\"LConn2\"]},\"type\":\"ConnectorPlacement.EquallySpacedRectSide\",\"uuid\":\"c872503a-61af-4937-bdf2-4de4f8645573\"},{\"content\":{\"connectorIds\":[\"RConn1\",\"RConn2\"],\"side\":\"RIGHT\"},\"type\":\"ConnectorPlacement.EquallySpacedRectSide\",\"uuid\":\"3b83f060-86a2-4569-84b5-d9f7c0485347\"},{\"content\":{\"connectorIds\":[\"In1\"],\"side\":\"TOP\"},\"type\":\"ConnectorPlacement.EquallySpacedRectSide\",\"uuid\":\"bf191d46-ce71-4d15-9dd0-24cc57253577\"}]},\"type\":\"ConnectorPlacement.EquallySpacedConnector\",\"uuid\":\"1b28ceee-25d0-45ae-a3c4-c2563f0d63ba\"}],\"packageUris\":[\"http://schema.mathworks.com/mf0/Connector/R2020b\"],\"version\":\"1.0\"}"
  full-bridge 2 : Subsystem
      settings: PortSchema="{\"entries\":[{\"content\":{\"sides\":[{\"content\":{\"connectorIds\":[\"LConn1\",\"LConn2\"]},\"type\":\"ConnectorPlacement.EquallySpacedRectSide\",\"uuid\":\"c872503a-61af-4937-bdf2-4de4f8645573\"},{\"content\":{\"connectorIds\":[\"RConn1\",\"RConn2\"],\"side\":\"RIGHT\"},\"type\":\"ConnectorPlacement.EquallySpacedRectSide\",\"uuid\":\"3b83f060-86a2-4569-84b5-d9f7c0485347\"},{\"content\":{\"connectorIds\":[\"In1\"],\"side\":\"TOP\"},\"type\":\"ConnectorPlacement.EquallySpacedRectSide\",\"uuid\":\"bf191d46-ce71-4d15-9dd0-24cc57253577\"}]},\"type\":\"ConnectorPlacement.EquallySpacedConnector\",\"uuid\":\"1b28ceee-25d0-45ae-a3c4-c2563f0d63ba\"}],\"packageUris\":[\"http://schema.mathworks.com/mf0/Connector/R2020b\"],\"version\":\"1.0\"}"
  single_phase_dab_transformer : Subsystem
  Udc(+) : PMIOPort  Side=Left
  udc(+) : PMIOPort  Port=2  Side=Right
  Udc(-) : PMIOPort  Port=3  Side=Left
  udc(-) : PMIOPort  Port=4  Side=Right
  tag scope: CFi_dc1_current_modB=global, dab_current_input_modB=global, dab_voltage_input_modB=global
  wires:
  Bus Selector1/1 -> full-bridge 2/1(gate_commands)
  Bus Selector/1 -> full-bridge 1/1(gate_commands)
  dab_gate_cmds/1 -> Bus Selector1/1, Bus Selector/1
  PS-Simulink Converter6/1 -> [dab_current_input_modB]  "idc"
  PS-Simulink Converter4/1 -> [dab_voltage_input_modB]  "udc1_dab_modA"
  PS-Simulink Converter1/1 -> [CFi_dc1_current_modB]  "CFi_dc_curren"
  connections:
  full-bridge 2/LConn2 -- single_phase_dab_transformer/RConn2
  full-bridge 2/LConn1 -- single_phase_dab_transformer/RConn1
  Current Sensor2/RConn1 -- PS-Simulink Converter6/LConn1
  Udc(+)/RConn1 -- Current Sensor2/LConn1
  Current Sensor2/RConn2 -- LFi_dc/LConn1
  full-bridge 2/RConn2 -- udc(-)/RConn1
  full-bridge 2/RConn1 -- udc(+)/RConn1
  full-bridge 1/LConn1 -- single_phase_dab_transformer/LConn1
  PS-Simulink Converter4/LConn1 -- Voltage Sensor/RConn1
  Current Sensor/RConn1 -- PS-Simulink Converter1/LConn1
  Current Sensor/LConn1 -- CFi_dc1/RConn1
  Udc(-)/RConn1 -- Voltage Sensor/RConn2 -- full-bridge 1/RConn2 -- Current Sensor/RConn2
  LFi_dc/RConn1 -- Voltage Sensor/LConn1 -- full-bridge 1/RConn1 -- CFi_dc1/LConn1
  full-bridge 1/LConn2 -- single_phase_dab_transformer/LConn2

== system sst_llc_npc_inv/dcdc_llc_modB/llc_ctrl ==
  dab_voltage&current_controllers : Subsystem
  modulator : Subsystem
  references : Subsystem
  sampling_i_filter1 : Subsystem
  sampling_v_filter1 : Subsystem
  sampling_v_filter2 : Subsystem
  dab_gate_cmds : Outport
  wires:
  references/1(vout_ref) -> sampling_v_filter2/1(in)
  sampling_v_filter2/1(out_pu) -> dab_voltage&current_controllers/3(dab_voltage_output pu_reference)  "dab_voltage_output_pu_reference"
  sampling_v_filter1/1(out_pu) -> dab_voltage&current_controllers/2(dab_voltage_output_pu)  "dab_voltage_output_pu"
  sampling_i_filter1/1(out_pu) -> dab_voltage&current_controllers/1(dab_current_input_pu)  "dab_current_input_pu"
  [dab_current_input_modB] -> sampling_i_filter1/1(in)
  [dab_voltage_output_modB] -> sampling_v_filter1/1(in)
  [TRGO_DCDC_2] -> dab_voltage&current_controllers/Trigger
  modulator/1(dab_gate_cmds) -> dab_gate_cmds/1
  [time_dab_module_2] -> dab_voltage&current_controllers/4(time_dab_module_2)  "time_dab_module_2"
  dab_voltage&current_controllers/1(freq_pu) -> modulator/1(freq_pu)
  dab_voltage&current_controllers/2(phase_disp) -> modulator/2(phase_displacement)
